simulink library "delay_ic_lib"  (R2016b)
settings: Solver=ode45  StartTime=0.0  StopTime=10.0  RelTol=1e-3  EnableMultiTasking=on
values from neighbouring files (symbols this model uses):
  ase_state_ic_A_B_ISS_ISS = single([0 0 0])    [ase_augmented_state_estimator_init.m]
  ase_state_ic_accel_bias = single([0 0 0])    [ase_augmented_state_estimator_init.m]
  ase_state_ic_aug_state_enum = uint8(0)    [ase_augmented_state_estimator_init.m]
  ase_state_ic_confidence = ase_status_converged    [ase_augmented_state_estimator_init.m]
  ase_state_ic_gyro_bias = single([0 0 0])    [ase_augmented_state_estimator_init.m]
  ase_state_ic_ml_P_cam_ISS_ISS = single([0 0 0])    [ase_augmented_state_estimator_init.m]
  ase_state_ic_ml_quat_ISS2cam = single([0 0 0 1])    [ase_augmented_state_estimator_init.m]
  ase_state_ic_status = ase_status_acquiring    [ase_augmented_state_estimator_init.m]
  tun_ase_state_ic_P_B_ISS_ISS = landmark_pos.Data(first_obs_row, :)    [ase_hw_data_test.m]
  tun_ase_state_ic_P_EST_ISS_ISS = tun_ase_state_ic_P_B_ISS_ISS + p_imu_body_iss    [ase_hw_data_test.m]
  tun_ase_state_ic_quat_ISS2B = landmark_quat.Data(first_obs_row, :)    [ase_hw_data_test.m]
undefined symbols (not defined in the file or in its folder): ase_state_ic_cov_diag, ase_state_ic_of_P_cam_ISS_ISS, ase_state_ic_of_quat_ISS2cam, ase_total_num_states, tun_ase_state_ic_cov_diag, tun_ase_state_ic_omega_B_ISS_B, tun_ase_state_ic_V_B_ISS_ISS, tun_aug_ic_cov
settings Model: Creator=jfusco1  LastModifiedBy=jfusco1
settings DataIOCC: LimitDataPoints=on  SaveFormat=Array
settings OptimizationCC: LifeSpan=inf
settings DebuggingCC: AllowSymbolicDim=off  SFUnexpectedBacktrackingDiag=warning  SFNoUnconditionalDefaultTransitionDiag=warning  SFExecutionAtInitializationDiag=none
settings HardwareCC: ProdBitPerPointer=32  ProdBitPerSizeT=32  ProdBitPerPtrDiffT=32  ProdLargestAtomicFloat=None  ProdIntDivRoundTo=Undefined  ProdEndianess=Unspecified  ProdWordSize=32  ProdHWDeviceType=32-bit Generic
settings ModelReferenceCC: PropagateSignalLabelsOutOfModel=off
settings GRTTargetCC: TargetLangStandard=C89/C90 (ANSI)  GeneratePreprocessorConditionals=Disable all
settings ConfigComp: CovMetricSettings=dw  CovHtmlReporting=on  CovSaveCumulativeToWorkspaceVar=on  CovSaveSingleToWorkspaceVar=on  CovExternalEMLEnable=off

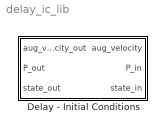
== system delay_ic_lib ==
  Delay - Initial Conditions : Subsystem

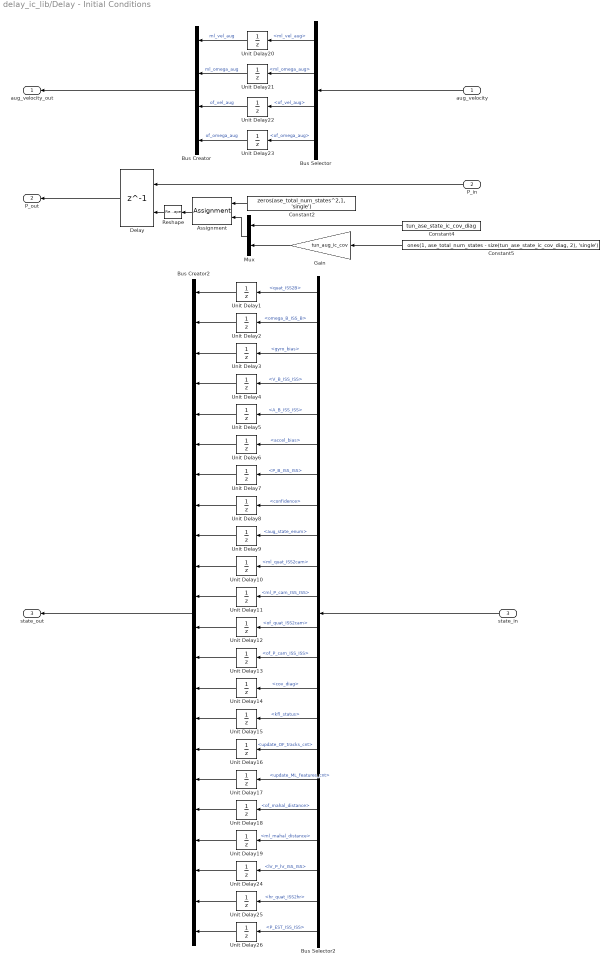
== system delay_ic_lib/Delay - Initial Conditions ==
  aug_velocity : Inport
  P_in : Inport  Port=2
  state_in : Inport  Port=3  OutDataTypeStr=Bus: kfl_msg
  Assignment : Assignment  DiagnosticForDimensions=Warning  IndexOptions=Index vector (dialog)  Indices=1:ase_total_num_states+1:ase_total_num_states^2  OutputSizes=1
  Bus Creator : BusCreator  Inputs=4
  Bus Creator2 : BusCreator  Inputs=22  OutDataTypeStr=Bus: kfl_msg  NonVirtualBus=on
      settings: InheritFromInputs=off
  Bus Selector : BusSelector  OutputSignals=ml_vel_aug,ml_omega_aug,of_vel_aug,of_omega_aug
  Bus Selector2 : BusSelector  OutputSignals=quat_ISS2B,omega_B_ISS_B,gyro_bias,V_B_ISS_ISS,A_B_ISS_ISS,accel_bias,P_B_ISS_ISS,confidence,aug_state_enum,ml_quat_ISS2cam,ml_P_cam_ISS_ISS,of_quat_ISS2cam,of_P_cam_ISS_ISS,cov_diag,kfl_status,update_OF_tracks_cnt,update_ML_features_cnt,of_mahal_distance,ml_mahal_distance,hr_P_hr_ISS_ISS,hr_quat_ISS2hr,P_EST_ISS_ISS
  Constant2 : Constant  Value=zeros(ase_total_num_states^2,1, 'single')
  Constant4 : Constant  Value=tun_ase_state_ic_cov_diag
  Constant5 : Constant  Value=ones(1, ase_total_num_states - size(tun_ase_state_ic_cov_diag, 2), 'single')
  Delay : Delay  DelayLength=1  InitialConditionSource=Input port  InitialCondition=0
      settings: InputPortMap=u0,p4
  Gain : Gain  Gain=tun_aug_ic_cov
  Mux : Mux  Inputs=2
  Reshape : Reshape  OutputDimensionality=Customize  OutputDimensions=[ase_total_num_states,ase_total_num_states]
  Unit Delay1 : UnitDelay  InitialCondition=tun_ase_state_ic_quat_ISS2B  SampleTime=-1
      settings: AttributesFormatString=IC: %<InitialCondition>
  Unit Delay10 : UnitDelay  InitialCondition=ase_state_ic_ml_quat_ISS2cam  SampleTime=-1
      settings: AttributesFormatString=IC: %<InitialCondition>
  Unit Delay11 : UnitDelay  InitialCondition=ase_state_ic_ml_P_cam_ISS_ISS  SampleTime=-1
      settings: AttributesFormatString=IC: %<InitialCondition>
  Unit Delay12 : UnitDelay  InitialCondition=ase_state_ic_of_quat_ISS2cam  SampleTime=-1
      settings: AttributesFormatString=IC: %<InitialCondition>
  Unit Delay13 : UnitDelay  InitialCondition=ase_state_ic_of_P_cam_ISS_ISS  SampleTime=-1
      settings: AttributesFormatString=IC: %<InitialCondition>
  Unit Delay14 : UnitDelay  InitialCondition=ase_state_ic_cov_diag  SampleTime=-1
      settings: AttributesFormatString=IC: %<InitialCondition>
  Unit Delay15 : UnitDelay  InitialCondition=ase_state_ic_status  SampleTime=-1
      settings: AttributesFormatString=IC: %<InitialCondition>
  Unit Delay{16..25} (10 alike) : UnitDelay  SampleTime=-1
      settings: AttributesFormatString=IC: %<InitialCondition>
  Unit Delay2 : UnitDelay  InitialCondition=tun_ase_state_ic_omega_B_ISS_B  SampleTime=-1
      settings: AttributesFormatString=IC: %<InitialCondition>
  Unit Delay26 : UnitDelay  InitialCondition=tun_ase_state_ic_P_EST_ISS_ISS  SampleTime=-1
      settings: AttributesFormatString=IC: %<InitialCondition>
  Unit Delay3 : UnitDelay  InitialCondition=ase_state_ic_gyro_bias  SampleTime=-1
      settings: AttributesFormatString=IC: %<InitialCondition>
  Unit Delay4 : UnitDelay  InitialCondition=tun_ase_state_ic_V_B_ISS_ISS  SampleTime=-1
      settings: AttributesFormatString=IC: %<InitialCondition>
  Unit Delay5 : UnitDelay  InitialCondition=ase_state_ic_A_B_ISS_ISS  SampleTime=-1
      settings: AttributesFormatString=IC: %<InitialCondition>
  Unit Delay6 : UnitDelay  InitialCondition=ase_state_ic_accel_bias  SampleTime=-1
      settings: AttributesFormatString=IC: %<InitialCondition>
  Unit Delay7 : UnitDelay  InitialCondition=tun_ase_state_ic_P_B_ISS_ISS  SampleTime=-1
      settings: AttributesFormatString=IC: %<InitialCondition>
  Unit Delay8 : UnitDelay  InitialCondition=ase_state_ic_confidence  SampleTime=-1
      settings: AttributesFormatString=IC: %<InitialCondition>
  Unit Delay9 : UnitDelay  InitialCondition=ase_state_ic_aug_state_enum  SampleTime=-1
      settings: AttributesFormatString=IC: %<InitialCondition>
  aug_velocity_out : Outport
  P_out : Outport  Port=2
  state_out : Outport  Port=3
  wires:
  Unit Delay24/1 -> Bus Creator2/20
  Bus Selector2/20 -> Unit Delay24/1  "<hr_P_hr_ISS_ISS>"
  Bus Selector2/21 -> Unit Delay25/1  "<hr_quat_ISS2hr>"
  Unit Delay25/1 -> Bus Creator2/21
  Bus Selector/4 -> Unit Delay23/1  "<of_omega_aug>"
  Bus Selector/3 -> Unit Delay22/1  "<of_vel_aug>"
  Bus Selector/2 -> Unit Delay21/1  "<ml_omega_aug>"
  Bus Selector/1 -> Unit Delay20/1  "<ml_vel_aug>"
  aug_velocity/1 -> Bus Selector/1
  Bus Creator/1 -> aug_velocity_out/1
  Unit Delay22/1 -> Bus Creator/3  "of_vel_aug"
  Unit Delay21/1 -> Bus Creator/2  "ml_omega_aug"
  Unit Delay23/1 -> Bus Creator/4  "of_omega_aug"
  Unit Delay20/1 -> Bus Creator/1  "ml_vel_aug"
  Unit Delay19/1 -> Bus Creator2/19
  Unit Delay18/1 -> Bus Creator2/18
  Bus Selector2/19 -> Unit Delay19/1  "<ml_mahal_distance>"
  Bus Selector2/18 -> Unit Delay18/1  "<of_mahal_distance>"
  Unit Delay9/1 -> Bus Creator2/9
  Unit Delay5/1 -> Bus Creator2/5
  Unit Delay12/1 -> Bus Creator2/12
  Unit Delay3/1 -> Bus Creator2/3
  Unit Delay6/1 -> Bus Creator2/6
  Unit Delay7/1 -> Bus Creator2/7
  Unit Delay8/1 -> Bus Creator2/8
  Unit Delay10/1 -> Bus Creator2/10
  Unit Delay11/1 -> Bus Creator2/11
  Unit Delay4/1 -> Bus Creator2/4
  Bus Selector2/12 -> Unit Delay12/1  "<of_quat_ISS2cam>"
  Bus Selector2/11 -> Unit Delay11/1  "<ml_P_cam_ISS_ISS>"
  Bus Selector2/10 -> Unit Delay10/1  "<ml_quat_ISS2cam>"
  Bus Selector2/9 -> Unit Delay9/1  "<aug_state_enum>"
  Bus Selector2/8 -> Unit Delay8/1  "<confidence>"
  Bus Selector2/7 -> Unit Delay7/1  "<P_B_ISS_ISS>"
  Bus Selector2/6 -> Unit Delay6/1  "<accel_bias>"
  Bus Selector2/4 -> Unit Delay4/1  "<V_B_ISS_ISS>"
  Bus Selector2/5 -> Unit Delay5/1  "<A_B_ISS_ISS>"
  Unit Delay2/1 -> Bus Creator2/2
  Bus Selector2/3 -> Unit Delay3/1  "<gyro_bias>"
  Unit Delay1/1 -> Bus Creator2/1
  Bus Selector2/2 -> Unit Delay2/1  "<omega_B_ISS_B>"
  Bus Selector2/1 -> Unit Delay1/1  "<quat_ISS2B>"
  Bus Creator2/1 -> state_out/1
  Bus Selector2/13 -> Unit Delay13/1  "<of_P_cam_ISS_ISS>"
  Bus Selector2/15 -> Unit Delay15/1  "<kfl_status>"
  Bus Selector2/14 -> Unit Delay14/1  "<cov_diag>"
  Unit Delay14/1 -> Bus Creator2/14
  Unit Delay15/1 -> Bus Creator2/15
  Unit Delay13/1 -> Bus Creator2/13
  state_in/1 -> Bus Selector2/1
  Bus Selector2/17 -> Unit Delay17/1  "<update_ML_features_cnt>"
  Unit Delay17/1 -> Bus Creator2/17
  Bus Selector2/16 -> Unit Delay16/1  "<update_OF_tracks_cnt>"
  Unit Delay16/1 -> Bus Creator2/16
  Bus Selector2/22 -> Unit Delay26/1  "<P_EST_ISS_ISS>"
  Unit Delay26/1 -> Bus Creator2/22
  P_in/1 -> Delay/1
  Constant2/1 -> Assignment/1
  Assignment/1 -> Reshape/1
  Mux/1 -> Assignment/2
  Constant4/1 -> Mux/1
  Gain/1 -> Mux/2
  Constant5/1 -> Gain/1
  Reshape/1 -> Delay/2
  Delay/1 -> P_out/1
